simulink model "trigger_test"  (Simulink 9.0)
settings: Solver=FixedStepDiscrete  StartTime=0.0  StopTime=1  FixedStep=1.000000  MaxStep=1  RelTol=1e-3  EnableMultiTasking=on
settings Model: SuppressorTable=22 serialization::archive 11 0 6 0 0 0 0 0  Creator=arnaud  LastModifiedBy=hbourbou
settings DataIOCC: ExternalInput=xin  LimitDataPoints=on  SaveFormat=StructureWithTime
settings DebuggingCC: UnderspecifiedInitializationDetection=Simplified  MergeDetectMultiDrivingBlocksExec=error  SolverPrmCheckMsg=warning
settings GRTTargetCC: GeneratePreprocessorConditionals=Disable all
settings ConfigComp: CovSFcnEnable=off

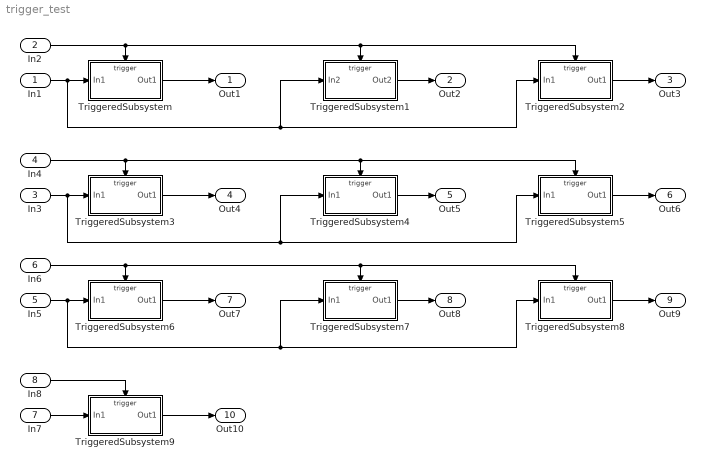
== system trigger_test ==
  In1 : Inport
  In2 : Inport  Port=2  OutDataTypeStr=boolean
  In3 : Inport  Port=3
  In4 : Inport  Port=4  OutDataTypeStr=int8
  In5 : Inport  Port=5
  In6 : Inport  Port=6  OutDataTypeStr=double
  In7 : Inport  Port=7  PortDimensions=3
  In8 : Inport  Port=8  OutDataTypeStr=boolean
  TriggeredSubsystem : Subsystem  TreatAsAtomicUnit=on
  TriggeredSubsystem1 : Subsystem  TreatAsAtomicUnit=on
  TriggeredSubsystem2 : Subsystem  TreatAsAtomicUnit=on
  TriggeredSubsystem3 : Subsystem  TreatAsAtomicUnit=on
  TriggeredSubsystem4 : Subsystem  TreatAsAtomicUnit=on
  TriggeredSubsystem5 : Subsystem  TreatAsAtomicUnit=on
  TriggeredSubsystem6 : Subsystem  TreatAsAtomicUnit=on
  TriggeredSubsystem7 : Subsystem  TreatAsAtomicUnit=on
  TriggeredSubsystem8 : Subsystem  TreatAsAtomicUnit=on
  TriggeredSubsystem9 : Subsystem  TreatAsAtomicUnit=on
  Out1 : Outport
  Out2 : Outport  Port=2
  Out3 : Outport  Port=3
  Out4 : Outport  Port=4
  Out5 : Outport  Port=5
  Out6 : Outport  Port=6
  Out7 : Outport  Port=7
  Out8 : Outport  Port=8
  Out9 : Outport  Port=9
  Out10 : Outport  Port=10
  wires:
  In1/1 -> TriggeredSubsystem2/1(In1), TriggeredSubsystem1/1(In2), TriggeredSubsystem/1(In1)
  In2/1 -> TriggeredSubsystem2/Trigger, TriggeredSubsystem1/Trigger, TriggeredSubsystem/Trigger
  TriggeredSubsystem/1(Out1) -> Out1/1
  TriggeredSubsystem1/1(Out2) -> Out2/1
  TriggeredSubsystem2/1(Out1) -> Out3/1
  In3/1 -> TriggeredSubsystem5/1(In1), TriggeredSubsystem4/1(In1), TriggeredSubsystem3/1(In1)
  In4/1 -> TriggeredSubsystem5/Trigger, TriggeredSubsystem4/Trigger, TriggeredSubsystem3/Trigger
  TriggeredSubsystem3/1(Out1) -> Out4/1
  TriggeredSubsystem4/1(Out1) -> Out5/1
  TriggeredSubsystem5/1(Out1) -> Out6/1
  In5/1 -> TriggeredSubsystem8/1(In1), TriggeredSubsystem7/1(In1), TriggeredSubsystem6/1(In1)
  In6/1 -> TriggeredSubsystem8/Trigger, TriggeredSubsystem7/Trigger, TriggeredSubsystem6/Trigger
  TriggeredSubsystem6/1(Out1) -> Out7/1
  TriggeredSubsystem7/1(Out1) -> Out8/1
  TriggeredSubsystem8/1(Out1) -> Out9/1
  In7/1 -> TriggeredSubsystem9/1(In1)
  In8/1 -> TriggeredSubsystem9/Trigger
  TriggeredSubsystem9/1(Out1) -> Out10/1

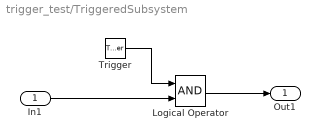
== system trigger_test/TriggeredSubsystem ==
  In1 : Inport
  Trigger : TriggerPort  VariantControl=(inherit)  ShowOutputPort=on  PortDimensions=1
  Logical Operator : Logic  AllPortsSameDT=off  OutDataTypeStr=boolean
  Out1 : Outport
  wires:
  Trigger/1 -> Logical Operator/1
  In1/1 -> Logical Operator/2
  Logical Operator/1 -> Out1/1

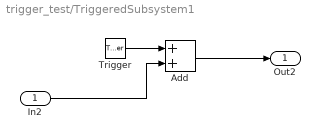
== system trigger_test/TriggeredSubsystem1 ==
  In2 : Inport
  Trigger : TriggerPort  TriggerType=falling  VariantControl=(inherit)  ShowOutputPort=on  PortDimensions=1
  Add : Sum
  Out2 : Outport
  wires:
  Trigger/1 -> Add/1
  In2/1 -> Add/2
  Add/1 -> Out2/1

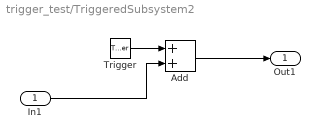
== system trigger_test/TriggeredSubsystem2 ==
  In1 : Inport
  Trigger : TriggerPort  TriggerType=either  VariantControl=(inherit)  ShowOutputPort=on  PortDimensions=1
  Add : Sum
  Out1 : Outport
  wires:
  Trigger/1 -> Add/1
  In1/1 -> Add/2
  Add/1 -> Out1/1

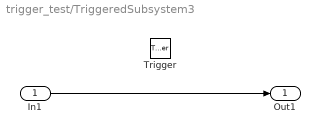
== system trigger_test/TriggeredSubsystem3 ==
  In1 : Inport
  Trigger : TriggerPort  VariantControl=(inherit)  PortDimensions=1
  Out1 : Outport
  wires:
  In1/1 -> Out1/1

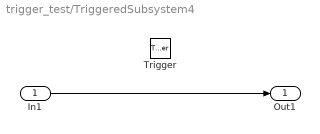
== system trigger_test/TriggeredSubsystem4 ==
  In1 : Inport
  Trigger : TriggerPort  TriggerType=falling  VariantControl=(inherit)  PortDimensions=1
  Out1 : Outport
  wires:
  In1/1 -> Out1/1

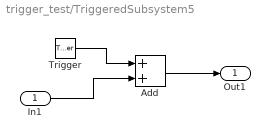
== system trigger_test/TriggeredSubsystem5 ==
  In1 : Inport
  Trigger : TriggerPort  TriggerType=either  VariantControl=(inherit)  ShowOutputPort=on  PortDimensions=1
  Add : Sum
  Out1 : Outport
  wires:
  Trigger/1 -> Add/1
  In1/1 -> Add/2
  Add/1 -> Out1/1

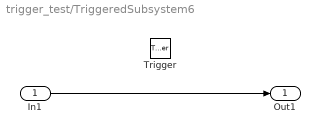
== system trigger_test/TriggeredSubsystem6 ==
  In1 : Inport
  Trigger : TriggerPort  VariantControl=(inherit)  PortDimensions=1
  Out1 : Outport
  wires:
  In1/1 -> Out1/1

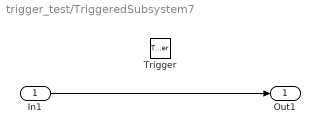
== system trigger_test/TriggeredSubsystem7 ==
  In1 : Inport
  Trigger : TriggerPort  TriggerType=falling  VariantControl=(inherit)  PortDimensions=1
  Out1 : Outport
  wires:
  In1/1 -> Out1/1

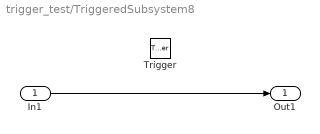
== system trigger_test/TriggeredSubsystem8 ==
  In1 : Inport
  Trigger : TriggerPort  TriggerType=either  VariantControl=(inherit)  PortDimensions=1
  Out1 : Outport
  wires:
  In1/1 -> Out1/1

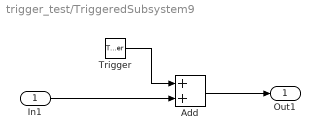
== system trigger_test/TriggeredSubsystem9 ==
  In1 : Inport
  Trigger : TriggerPort  TriggerType=either  VariantControl=(inherit)  ShowOutputPort=on  PortDimensions=1
  Add : Sum
  Out1 : Outport
  wires:
  Trigger/1 -> Add/1
  In1/1 -> Add/2
  Add/1 -> Out1/1
